simulink model "crob"  (Simulink 7.1)
settings: Solver=ode45  StartTime=0.0  StopTime=8  RelTol=1e-2
undefined symbols (not defined in the file or in its folder): gravedad, Kd, Kp
libraries: roblocks x2
settings Model: Creator=Hads  LastModifiedBy=Hads

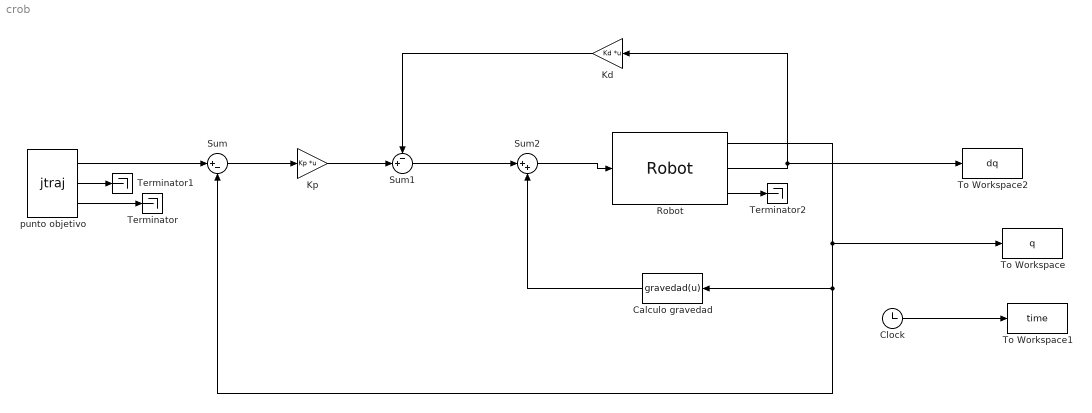
== system crob ==
  Calculo gravedad : MATLABFcn  Orientation=left  MATLABFcn=gravedad(u)
  Clock : Clock
      settings: Decimation=10
  Kd : Gain  Orientation=left  Gain=Kd  Multiplication=Matrix(K*u)  ParameterDataType=sfix(16)  ParameterScaling=2^0  OutDataType=sfix(16)  OutScaling=2^0
  Kp : Gain  Gain=Kp  Multiplication=Matrix(K*u)  ParameterDataType=sfix(16)  ParameterScaling=2^0  OutDataType=sfix(16)  OutScaling=2^0
  Robot : roblocks/Robot  SystemSampleTime=-1  robot=p560  q0=[0 0 0 0 0 0]
      link override Integrator1: InitialCondition=q0
  Sum : Sum  Inputs=|+-  OutDataType=sfix(16)  OutScaling=2^0
  Sum1 : Sum  Inputs=-+|  OutDataType=sfix(16)  OutScaling=2^0
  Sum2 : Sum  Inputs=|++  OutDataType=sfix(16)  OutScaling=2^0
  Terminator : Terminator
  Terminator1 : Terminator
  Terminator2 : Terminator
  To Workspace : ToWorkspace  VariableName=q  SampleTime=-1  SaveFormat=Array
  To Workspace1 : ToWorkspace  VariableName=time  SampleTime=-1  SaveFormat=Array
  To Workspace2 : ToWorkspace  VariableName=dq  SampleTime=-1  SaveFormat=Array
  punto objetivo : roblocks/jtraj  SystemSampleTime=-1  q0=[1 1 1 1 1 1]  qf=[1 1 1 1 1 1]  tmax=8
  wires:
  Sum/1 -> Kp/1
  Kp/1 -> Sum1/2
  Robot/1 -> To Workspace/1, Sum/2, Calculo gravedad/1
  Robot/2 -> Kd/1, To Workspace2/1
  Kd/1 -> Sum1/1
  Sum1/1 -> Sum2/1
  Sum2/1 -> Robot/1
  punto objetivo/1 -> Sum/1
  Clock/1 -> To Workspace1/1
  Calculo gravedad/1 -> Sum2/2
  punto objetivo/3 -> Terminator/1
  punto objetivo/2 -> Terminator1/1
  Robot/3 -> Terminator2/1
